simulink model "Arizona_base_GOAT"  (R2022a)
settings: Solver=FixedStepDiscrete  StartTime=0.0  StopTime=inf  FixedStep=Ts  RelTol=1e-3  EnableMultiTasking=on
undefined symbols (not defined in the file): DiscIntNeverNeededParam, Ended, IO307, N_Init, Nref, phi_Init, Single, x_Init, y_Init
libraries: speedgoatlib_fpga_dio x30, speedgoatlib_fpga_quadrature x19, simulink x10, speedgoatlib_IO141 x9, xpcobsoletelib x7, speedgoatlib_fpga x3, cstblocks x3
(part 3 of 3)

== stateflow chart Arizona_base_GOAT/Safety/Supervisor ==
  state evaluateSatefy
    state gantryAirbag [parallel]
      settings: executionOrder=3
      state defaultState
        exit:
        enableAirbags = true;
      state backAirbag
        entry:
        current_gantryAirbag = -5;
      state frontAirbag
        entry:
        current_gantryAirbag = 5;
      state stop_gantryAirbag
        entry:
        current_gantryAirbag = 0;
      (default) -> evaluateSatefy.gantryAirbag.defaultState
      evaluateSatefy.gantryAirbag.defaultState -> frontAirbag [order 1] : [homingDone && xNom<0.1075-xInit_end]
      evaluateSatefy.gantryAirbag.defaultState -> backAirbag [order 2] : [homingDone && xNom>1.035-xInit_end-0.1075]
      backAirbag -> stop_gantryAirbag : [velocity_x<=0]
      frontAirbag -> stop_gantryAirbag : [velocity_x>=0]
    state errorAirbag [parallel]
      settings: executionOrder=1
      state defaultState
      state errorStop
        entry:
        enableAirbags = true;
      (default) -> evaluateSatefy.errorAirbag.defaultState
      evaluateSatefy.errorAirbag.defaultState -> errorStop : [abs(error_x)>0.05 || abs(error_y)>0.05 || abs(error_phi)>0.05 || abs(phi)>atan(.01/2.6)]
    state carriageAirbag [parallel]
      settings: executionOrder=2
      state defaultState
        exit:
        enableAirbags = true;
      state leftAirbag
        entry:
        current_carriageAirbag = 5;
      state rightAirbag
        entry:
        current_carriageAirbag = -5;
      state stop_carriageAirbag
        entry:
        current_carriageAirbag = 0;
      (default) -> evaluateSatefy.carriageAirbag.defaultState
      evaluateSatefy.carriageAirbag.defaultState -> leftAirbag [order 1] : [homingDone && yNom<0.19-yInit_end]
      evaluateSatefy.carriageAirbag.defaultState -> rightAirbag [order 2] : [homingDone && yNom>3.2-yInit_end-0.19]
      leftAirbag -> stop_carriageAirbag : [velocity_y>=0]
      rightAirbag -> stop_carriageAirbag : [velocity_y<=0]
  state stopCarriage
    entry:
    stopSimulation = true;
  (default) -> evaluateSatefy
  evaluateSatefy -> stopCarriage : % Stop simulation if the airbags are active with zero current and the velocity is small.
      | [ enableAirbags && current_carriageAirbag == 0 && current_gantryAirbag == 0 && sqrt(velocity_x^2+velocity_y^2)<0.01 ]
  data: xInit_end constant double =x_Init(end); yInit_end constant double =y_Init(end); homingDone input double; error_y input double =false; yNom input double =false; velocity_y input double =false; error_x input double =false; current_carriageAirbag output double =0; enableAirbags output double =false; xNom input double =false; velocity_x input double =false; error_phi input double =false; current_gantryAirbag output double =0; stopSimulation output double =false; phi input double

== stateflow chart Arizona_base_GOAT/Penholder mechanism1/Change color Chart ==
  state MOVE_PENHOLDER
    state MAIN [parallel]
      settings: executionOrder=1
      state INITIAL
        entry:
        active=0;
        job=0;
      state IDLE
      state HOMING
      state FINISHED
        entry:
        active=0;
      state GOING_UP
        entry:
        active=1;
      state GOING_DOWN
        entry:
        active=1;
      state ROTATING
      (default) -> MOVE_PENHOLDER.MAIN.INITIAL
      MOVE_PENHOLDER.MAIN.IDLE -> MOVE_PENHOLDER.MAIN.IDLE [order 3] : [job~=change_color ...
          | && change_color==0]
          | {job=change_color}
      MOVE_PENHOLDER.MAIN.INITIAL -> MOVE_PENHOLDER.MAIN.IDLE
      MOVE_PENHOLDER.MAIN.IDLE -> GOING_UP [order 1] : [job ~= change_color && change_color~=0 ...
          | && homingDone ~=0 && change_color~=6]
          | {send(go_up,VERTICAL);job=change_color}
      MOVE_PENHOLDER.MAIN.IDLE -> HOMING [order 4] : [homingDone==0 ...
          | && change_color==5]
          | {send(start_homing,HOME)}
      FINISHED -> MOVE_PENHOLDER.MAIN.IDLE
      MOVE_PENHOLDER.MAIN.IDLE -> GOING_DOWN [order 2] : [job ~= change_color ...
          | && change_color==6]
          | {send(go_down,VERTICAL);job=change_color}
      HOMING -> FINISHED : [homing_done]
      GOING_UP -> FINISHED [order 1] : [is_up && job==5]
      GOING_DOWN -> FINISHED : [is_down]
      GOING_UP -> ROTATING [order 2] : [is_up && job~=5]
          | {send(start_rotate,ROTATION)}
      ROTATING -> GOING_DOWN : [rotate_done && job~=7]
          | {send(go_down,VERTICAL)}
    state VERTICAL [parallel]
      settings: executionOrder=2
      state ALREADY_DOWN
      state DOWN
        entry:
        jogspeed_Z=0;
      state MOVING_UP
        entry:
        jogspeed_Z=1;
      state MOVING_DOWN
        entry:
        jogspeed_Z=-1;
      state INITIAL
      state UP
        entry:
        jogspeed_Z=0;
      state ALREADY_UP
      ALREADY_DOWN -> DOWN : [after(0.1,sec)]{send(is_down,MAIN)}
      DOWN -> ALREADY_DOWN [order 2] : go_down
      DOWN -> MOVE_PENHOLDER.VERTICAL.MOVING_UP [order 1] : go_up
      MOVING_DOWN -> DOWN : [limitSwitch_z_down==1]
          | {send(is_down,MAIN)}
      (default) -> MOVE_PENHOLDER.VERTICAL.INITIAL
      MOVE_PENHOLDER.VERTICAL.INITIAL -> MOVE_PENHOLDER.VERTICAL.MOVING_UP [order 1] : go_up
      MOVE_PENHOLDER.VERTICAL.INITIAL -> MOVING_DOWN [order 2] : go_down
      MOVE_PENHOLDER.VERTICAL.UP -> MOVING_DOWN [order 1] : go_down
      MOVE_PENHOLDER.VERTICAL.MOVING_UP -> MOVE_PENHOLDER.VERTICAL.UP : [limitSwitch_z_up==1]
          | {send(is_up,MAIN)}
      ALREADY_UP -> MOVE_PENHOLDER.VERTICAL.UP : [after(0.1,sec)]{send(is_up,MAIN)}
      MOVE_PENHOLDER.VERTICAL.UP -> ALREADY_UP [order 2] : go_up
    state ROTATION [parallel]
      settings: executionOrder=3
      state INITIAL
        en: color_pos=1;
      state INITIALIZE
        entry:
        rot_change = change_color-color_pos;
      state IDLE
        entry:
        jogspeed_Theta=0;
      state CHECK_ROTATE
      state ARRIVAL
        entry:
        counter=counter-1*sign(counter);
        color_pos = change_color;
      state DEPARTURE
        entry:
        jogspeed_Theta = 1*sign(counter);
      (default) -> MOVE_PENHOLDER.ROTATION.INITIAL
      MOVE_PENHOLDER.ROTATION.INITIAL -> MOVE_PENHOLDER.ROTATION.IDLE : [after(0.1,sec)]
      MOVE_PENHOLDER.ROTATION.IDLE -> INITIALIZE : [start_rotate]
      INITIALIZE -> CHECK_ROTATE [order 1] : [-2<=rot_change && rot_change<=2]
          | {counter = rot_change}
      INITIALIZE -> CHECK_ROTATE [order 3] : [rot_change== 3]{counter =-1}
      INITIALIZE -> CHECK_ROTATE [order 2] : [rot_change==-3]{counter = 1}
      ARRIVAL -> MOVE_PENHOLDER.ROTATION.IDLE [order 1] : [counter==0 && change_color==7]
          | {send(rotate_done,MAIN); color_pos=1}
      ARRIVAL -> MOVE_PENHOLDER.ROTATION.IDLE [order 2] : [counter==0 && change_color~=7]
          | {send(rotate_done,MAIN)}
      CHECK_ROTATE -> DEPARTURE : [counter~=0]
      DEPARTURE -> ARRIVAL : [after(1,sec) && ...
          | limitSwitch_Theta==1]
      ARRIVAL -> DEPARTURE [order 3] : [counter~=0]
    state HOME [parallel]
      settings: executionOrder=4
      state MOVING_UP
        entry:
        jogspeed_Z=1;
      state INITIAL
      state UP
        entry:
        jogspeed_Z=0;
      state DONE
        entry:
        jogspeed_Theta=0;
      state ROTATE
        entry:
        jogspeed_Theta=1;
      (default) -> MOVE_PENHOLDER.HOME.INITIAL
      MOVE_PENHOLDER.HOME.INITIAL -> MOVE_PENHOLDER.HOME.MOVING_UP : [start_homing]
      DONE -> MOVE_PENHOLDER.HOME.INITIAL : {send(homing_done,MAIN)}
      MOVE_PENHOLDER.HOME.MOVING_UP -> MOVE_PENHOLDER.HOME.UP : [limitSwitch_z_up==1]
      MOVE_PENHOLDER.HOME.UP -> DONE [order 1] : [limitSwitch_Theta==1]
      MOVE_PENHOLDER.HOME.UP -> ROTATE [order 2] : [after(0.1,sec) ...
          | && limitSwitch_Theta~=1]
      ROTATE -> DONE : [after(0.1,sec) ...
          | && limitSwitch_Theta==1]
  (default) -> MOVE_PENHOLDER
  data: change_color input; limitSwitch_z_up input; limitSwitch_z_down input; limitSwitch_Theta input; jogspeed_Z output; jogspeed_Theta output; counter local; active output; job local; rot_change local; color_pos local; homingDone input
  events: is_down local FUNCTION_CALL_EVENT; is_up local FUNCTION_CALL_EVENT; go_up local FUNCTION_CALL_EVENT; go_down local FUNCTION_CALL_EVENT; start_rotate local FUNCTION_CALL_EVENT; rotate_done local FUNCTION_CALL_EVENT; start_homing local FUNCTION_CALL_EVENT; homing_done local FUNCTION_CALL_EVENT

== stateflow chart Arizona_base_GOAT/Trial control without penholder ==
  state Home
    en:
    homeTrigger = 1;
  state idle
    en:
    trialTrigger = 0;
    homeTrigger = 0;
  state trial
    en:
    trialTrigger = 1;
    timeIndex = 0;
    trialIndex++;
    du:
    timeIndex++;
  idle -> trial [order 2] : %Start ILC trial
      | [startTrial]
  Home -> idle : %Transition if home is completed.
      | [homingDone]
  idle -> Home [order 1] : %Redo homing during run.
      | [startHoming]
  trial -> idle : %Transition if trial is ended.
      | [TrialDone]
  (default) -> idle
  data: startHoming input; homeTrigger output double; homingDone input double; startTrial input double; startPenholder input; trialTrigger output double =0; timeIndex local double =0; trialIndex output double =0; TrialDone input; change_color output double; penholder_active input; PenColor input

== stateflow chart Arizona_base_GOAT/Trial control without penholder1 ==
  state initialization
    en:
    homeTrigger = 1;
  state idle
    en:
    trialTrigger = 0;
    homeTrigger =0;
  state trial
    en:
    trialTrigger = 1;
    timeIndex = 0;
    trialIndex++;
    du:
    timeIndex++;
  idle -> trial [order 2] : %Start ILC trial
      | [startTrial]
  initialization -> idle : %Transition if initialization is completed.
      | [homingDone]
  (default) -> initialization
  idle -> initialization [order 1] : %Redo homing during run.
      | [startHoming]
  trial -> idle : %Transition if trial is ended.
      | [TrialDone]
  data: startHoming input; homeTrigger output double; homingDone input double; startTrial input double; startPenholder input; trialTrigger output double =0; timeIndex local double =0; trialIndex output double =0; TrialDone input; change_color output double; penholder_active input; PenColor input

== stateflow chart Arizona_base_GOAT/Homing/Enabled subsystem/Reset/Supervisor ==
  state MOVE_PEN_UP
    entry:
    change_color=5;
  state PEN_READY
    entry:
    change_color=0;
  state MoveToLimitSwitches
    state reset_gantryLeft [parallel]
      settings: executionOrder=1
      state increase_jogspeed
        during:
        jogspeed_xL_reset = max(-0.10,jogspeed_xL_reset - 0.10*Ts/1);
      state stop
        entry:
        jogspeed_xL_reset = 0;
      (default) -> MoveToLimitSwitches.reset_gantryLeft.increase_jogspeed
      MoveToLimitSwitches.reset_gantryLeft.increase_jogspeed -> MoveToLimitSwitches.reset_gantryLeft.stop : [duration(limitswitch_xL) >= 0.01]
    state reset_gantryright [parallel]
      settings: executionOrder=2
      state increase_jogspeed
        during:
        jogspeed_xR_reset = max(-0.10,jogspeed_xR_reset - 0.10*Ts/1);
      state stop
        entry:
        jogspeed_xR_reset = 0;
      (default) -> MoveToLimitSwitches.reset_gantryright.increase_jogspeed
      MoveToLimitSwitches.reset_gantryright.increase_jogspeed -> MoveToLimitSwitches.reset_gantryright.stop : [duration(limitswitch_xR) >= 0.01]
    state reset_carriage [parallel]
      settings: executionOrder=3
      state increase_jogspeed
        during:
        jogspeed_y_reset = max(-0.25,jogspeed_y_reset - 0.25*Ts/1);
      state stop
        entry:
        jogspeed_y_reset = 0;
      (default) -> MoveToLimitSwitches.reset_carriage.increase_jogspeed
      MoveToLimitSwitches.reset_carriage.increase_jogspeed -> MoveToLimitSwitches.reset_carriage.stop : [duration(limitswitch_y) >= 0.01]
  state enablePointToRefs
    entry:
    resetDone = true;
  (default) -> MOVE_PEN_UP
  MOVE_PEN_UP -> PEN_READY : [after(1,sec) && penholder_active==0]
  PEN_READY -> MoveToLimitSwitches
  MoveToLimitSwitches -> enablePointToRefs : [(jogspeed_xL_reset==0) && (jogspeed_xR_reset==0) && (jogspeed_y_reset==0)]
  data: jogspeed_y_reset output double =-0.25*Ts/1; jogspeed_xL_reset output double =-0.10*Ts/1; limitswitch_y input double; limitswitch_xL input double; limitswitch_xR input double; jogspeed_xR_reset output double =-0.10*Ts/1; resetDone output double =0; Ts local double =Ts; penholder_active input; change_color output double
